simulink model "Ejer4_EcLotkaVolterra"  (R2023b)
settings: Solver=VariableStepAuto  StartTime=0.0  StopTime=10.0  RelTol=1e-3
values from neighbouring files (symbols this model uses):
  a = 2.7    [EjerciciosModelosContinuos.m]
  b = 0.7    [EjerciciosModelosContinuos.m]
settings Model: Creator=alfre  LastModifiedBy=alfre

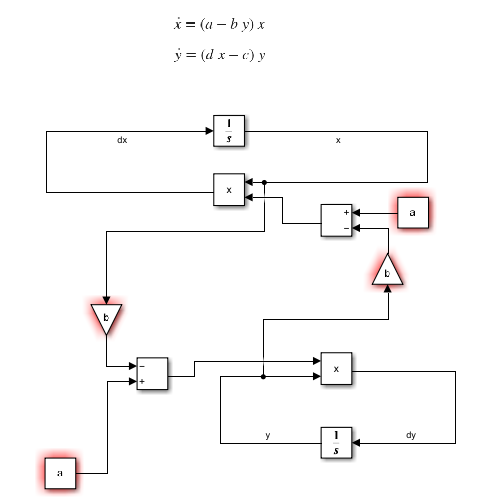
[thumbnail: Simulink's stored preview of the top-level diagram]
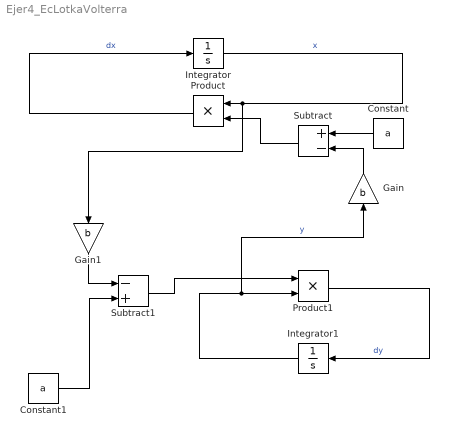
== system Ejer4_EcLotkaVolterra ==
  Constant : Constant  Value=a
  Constant1 : Constant  Value=a
  Gain : Gain  Gain=b
  Gain1 : Gain  Gain=b
  Integrator : Integrator
  Integrator1 : Integrator
  Product : Product
  Product1 : Product
  Subtract : Sum  Inputs=+-
  Subtract1 : Sum  Inputs=-+
  wires:
  Product/1 -> Integrator/1  "dx"
  Integrator/1 -> Gain1/1, Product/1  "x"
  Constant/1 -> Subtract/1
  Subtract/1 -> Product/2
  Gain/1 -> Subtract/2
  Gain1/1 -> Subtract1/1
  Constant1/1 -> Subtract1/2
  Integrator1/1 -> Product1/2, Gain/1  "y"
  Subtract1/1 -> Product1/1
  Product1/1 -> Integrator1/1  "dy"
